simulink model "RHONN_EKF_FEEDBACK_FINAL_28_JULIO_2021"  (R2017b)
settings: Solver=ode1  StartTime=0.0  StopTime=60  FixedStep=0.001  RelTol=1e-3
model workspace (MATLAB code in the model file):
  | % ESTADOS INICIALES DE LOS ESTADOS X1, X2 Y X3
  | % Donde:
  | % x1 es representado con un vector de 3x1.
  | % x2 es representado con un vector de 2x1.
  | % x3 es representado con un vector de 2x1.
  | 
  | % Definir estados iniciales de las variables x11, x12 y x13 respectivamente.
  | init_x11 = 0;
  | init_x12 = 0;
  | init_x13 = 0;
  | % Estado inicial de x1
  | init_state_x1 = [init_x11; init_x12; init_x13];
  | 
  | % Definir estados iniciales de las variables x21 y x22 respectivamente.
  | init_x21 = 0.1;
  | init_x22 = 0.1;
  | % Estado inicial de x2
  | init_state_x2 = [init_x21; init_x22];
  | 
  | % Definir estados iniciales de las variables x31 y x32 respectivamente.
  | init_x31 = 0.1;
  | init_x32 = 0.1;
  | % Estado inicial de x3
  | init_state_x3 = [init_x31; init_x32];
  | 
  | % Definir el estado inicial de la ley de control U, representado por un vector de 2x1.
  | init_U1 = -1;
  | init_U2 = -1;
  | init_U = [init_U1; init_U2];
  | 
  | % INICIALIZACION DE VARIABLES >>>>>>>>>>>>>>>>>>>>>>>>>>>>>>>>
  | 
  |     %Constantes iniciales
  |     %La mitad del ancho del robot mobil.
  |     R = 0.75;
  |     %La distancia del centro de Pc del robot mobil a la mitad del punto medio
  |     %de P0 en medio de las ruedas izquierda y derecha.
  |     d = 0.3;
  |     %Radio de la rueda.
  |     r = 0.15;
  |     %Masa del cuerpo.
  |     mc = 30;
  |     %Masa de la rueda con motor.
  |     mw = 1;
  |     %Ic,Iw,Im son los momentos de inercia del cuerpo sobre el eje vertical a
  |     %traves de Pc.
  |     Ic = 15.625;
  |     Iw = 0.005;
  |     Im = 0.0025;
  |     %Resistencia.
  |     Ra = diag([2.5,2.5]);
  |     %Inductancia.
  |     La = diag([0.048,0.048]);
  |     %Coeficiente de fuera electromotriz trasero.
  |     KE = diag([0.02,0.02]);
  |     %Relacion de transmision.
  |     N = diag([62.55,62.55]);
  |     %Constante de torque del motor.
  |     KT = diag([0.2613,0.2613]);
  |     %d11, d12 son los coeficientes de amortiguamiento.
  |     d11 = 0.5;
  |     d12 = d11;
  |     %>>>>>>>>>>>>>>>>>>>>>>>>>>>>>>>>>>>>>>>>>>>>>>>>>>>>>>>><
  | 
  |     m = mc + (2 * mw);
  |     I = (mc * (d ^ 2)) + (2 * mw * (R^2)) + Ic + (2*Im);
  |     m11 = 0.25 * ( R ^ -2 ) * (r ^ 2) * ((m * (R ^ 2)) + I) + Iw;
  |     m12 = 0.25 * ( R ^ -2 ) * (r ^ 2) * ((m * (R ^ 2)) - I);
  |     M = [m11, m12; m12, m11];
  |     D = diag([d11, d12]);
  | 
  | 
  |  %VALORES HUERISTICOS SEGUN EL PAPER
  | %MODELO MATEMATICO
  | 
  | 
  | %Constantes iniciales
  | %La mitad del ancho del robot mobil.
  | R = 0.75;
  | %La distancia del centro de Pc del robot mobil a la mitad del punto medio
  | %de P0 en medio de las ruedas izquierda y derecha.
  | d = 0.3;
  | %Radio de la rueda.
  | r = 0.15;
  | %Masa del cuerpo.
  | mc = 30;
  | %Masa de la rueda con motor.
  | mw = 1;
  | %Ic,Iw,Im son los momentos de inercia del cuerpo sobre el eje vertical a
  | %traves de Pc.
  | Ic = 15.625;
  | Iw = 0.005;
  | Im = 0.0025;
  | %Resistencia.
  | Ra = diag([2.5,2.5]);
  | %Inductancia.
  | La = diag([0.048,0.048]);
  | %Coeficiente de fuera electromotriz trasero.
  | KE = diag([0.02,0.02]);
  | %Relacion de transmision.
  | N = diag([62.55,62.55]);
  | %Constante de torque del motor.
  | KT = diag([0.2613,0.2613]);
  | %d11, d12 son los coeficientes de amortiguamiento.
  | d11 = 0.5;
  | d12 = d11;
  | 
  | 
  | 
  | %NOTA : los valores cuya definicion se encuentre en minuscula
  | %se utiliza para generar de manera dinamica con programacion
  | %la variable final que se utiliza en el programa.
  | %De manera que si llegara a ser necesario solo se modificarian las variables iniciales
  | 
  | %VARIABLES INICIALES ========================================
  | 
  | p1 = 1 * (10^8);
  | p2 = 1 * (10^2);
  | p3 = 1 * (10^8);
  | p4 = 1 * (10^2);
  | p5 = 1 * (10^2);
  | p6 = 1 * (10^2);
  | p7 = 1 * (10^2);
  | 
  | r1 = 1 * (10^4);
  | r2 = 5 * (10^4);
  | r3 = 1 * (10^4);
  | r4 = 1 * (10^1);
  | r5 = 1 * (10^1);
  | r6 = 1 * (10^3);
  | r7 = 1 * (10^3);
  | 
  | q1 = 5 * (10^5);
  | q2 = 5 * (10^5);
  | q3 = 5 * (10^5);
  | q4 = 1 * (10^1);
  | q5 = 1 * (10^1);
  | q6 = 1 * (10^3);
  | q7 = 1 * (10^3);
  | 
  | G1 = 0.00001;
  | G2 = 0.00001;
  | 
  | %VALOREES INICIALES DE LOS PESOS USADOS EN EKF
  | 
  | %PESOS DE W1
  | W11 = 0.1;
  | W12 = 0.1;
  | %PESOS DE W2
  | W21 = 0.1;
  | W22 = 0.1;
  | %PESOS DE W3
  | W31 = 0.1;
  | W32 = 0.1;
  | %PESOS DE W4
  | W41 = 0.1;
  | W42 = 0.1;
  | W43 = 0.1;
  | W44 = 0.1;
  | %PESOS DE W5
  | W51 = 0.1;
  | W52 = 0.1;
  | W53 = 0.1;
  | W54 = 0.1;
  | %PESOS DE W6
  | W61 = 0.1;
  | W62 = 0.1;
  | W63 = 0.1;
  | W64 = 0.1;
  | %PESOS DE W7
  | W71 = 0.1;
  | W72 = 0.1;
  | W73 = 0.1;
  | W74 = 0.1;
  | 
  | %VALOR DE LAS SIGMOIDALES SUAVES
  | B = 2 * exp(-3);    %Este valor debe ser mayor a cero pero en base a mis observaciones menor a 1.
  | FO = 1;   %Este valor es obtenido de la tesis de la Dra Alma debe ser CERCANO y MENOR a 1, si este se vuelve 1 funcionara como FKE unicamente
  | 
  | 
  | %VARIABLES FINALES ========================================
  | 
  | %PARAMETROS DE ENTRENAMIENTO EKF PARA RHONN 1
  | W1 = [W11; W12]; %VALOR INICIAL de Vector de pesos para x1
  | P1 = diag([p1, p1]); %VALOR INICIAL de Matriz diagonal inicial de P1
  | R1 = r1; % Valor de R1
  | Q1 = diag([q1, q1]); % Valor de Q1
  | 
  | %PARAMETROS DE ENTRENAMIENTO EKF PARA RHONN 2
  | W2 = [W21; W22]; %VALOR INICIAL de Vector de pesos para x2
  | P2 = diag([p2, p2]); %VALOR INICIAL de Matriz diagonal inicial de P2
  | R2 = r2; % Valor de R2
  | Q2 = diag([q2, q2]); % Valor de Q2
  | 
  | %PARAMETROS DE ENTRENAMIENTO EKF PARA RHONN 3
  | W3 = [W31; W32]; %VALOR INICIAL de Vector de pesos para x3
  | P3 = diag([p3, p3]); %VALOR INICIAL de Matriz diagonal inicial de P3
  | R3 = r3; % Valor de R3
  | Q3 = diag([q3, q3]); % Valor de Q3
  | 
  | %PARAMETROS DE ENTRENAMIENTO EKF PARA RHONN 4
  | W4 = [W41; W42; W43; W44]; %VALOR INICIAL de Vector de pesos para x4
  | P4 = diag([p4, p4, p4, p4]); %VALOR INICIAL de Matriz diagonal inicial de P4
  | R4 = r4; % Valor de R4
  | Q4 = diag([q4, q4, q4, q4]); % Valor de Q4
  | 
  | %PARAMETROS DE ENTRENAMIENTO EKF PARA RHONN 5
  | W5 = [W51; W52; W53; W54]; %VALOR INICIAL de Vector de pesos para x5
  | P5 = diag([p5, p5, p5, p5]); %VALOR INICIAL de Matriz diagonal inicial de P5
  | R5 = r5; % Valor de R5
  | Q5 = diag([q5, q5, q5, q5]); % Valor de Q5
  | 
  | %PARAMETROS DE ENTRENAMIENTO EKF PARA RHONN 6
  | W6 = [W61; W62; W63; W64]; %VALOR INICIAL de Vector de pesos para x6
  | P6 = diag([p6, p6, p6, p6]); %VALOR INICIAL de Matriz diagonal inicial de P6
  | R6 = r6; % Valor de R6
  | Q6 = diag([q6, q6, q6, q6]); % Valor de Q6
  | 
  | %PARAMETROS DE ENTRENAMIENTO EKF PARA RHONN 7
  | W7 = [W71; W72; W73; W74]; %VALOR INICIAL de Vector de pesos para x7
  | P7 = diag([p7, p7, p7, p7]); %VALOR INICIAL de Matriz diagonal inicial de P7
  | R7 = r7; % Valor de R7
  | Q7 = diag([q7, q7, q7, q7]); % Valor de Q7
  | 
  | 
  | % PARAMETROS DEL CONTROL POR RETROALIMENTACION
  | % Donde K1 es representado con una matriz diagonal 3x3
  | % Donde K2 es representado con una matriz diagonal 2x2
  | % Donde K3 es representado con una matriz diagonal 2x2
  | 
  | % Ganancias individuales de la diagonal K1
  | k11 = 70;
  | k12 = k11;
  | k13 = k11;
  | 
  | % Ganancias individuales de la diagonal K2.
  | k21 = 50;
  | k22 = k21;
  | 
  | % Ganancias individuales de la diagonal K3.
  | k31 = 200;
  | k32 = k31;
  | 
  | % Matrices de gananciasK1, K2, K3.
  | K1 = diag([k11, k12, k13]);
  | K2 = diag([k21, k22]);
  | K3 = diag([k31, k32]);
libraries: simulink x5
(part 1 of 2)
settings Model: Creator=52324  LastModifiedBy=52324

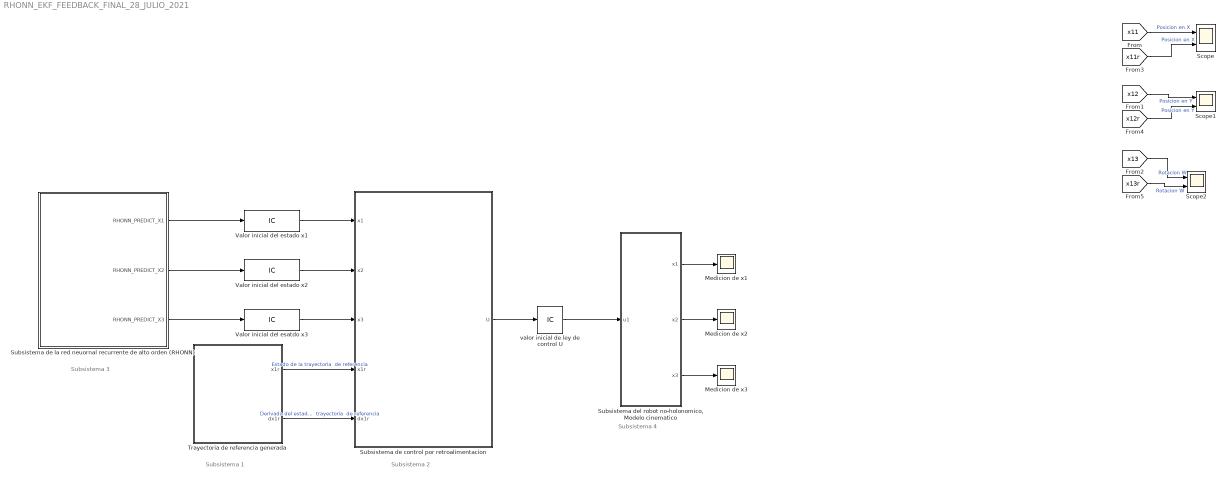
== system RHONN_EKF_FEEDBACK_FINAL_28_JULIO_2021 ==
  note: Subsistema 1
  note: Subsistema 2
  note: Subsistema 3
  note: Subsistema 4
  Medicion de x1 : Scope
  Medicion de x2 : Scope
  Medicion de x3 : Scope
  Scope : Scope  NumInputPorts=2
  Scope1 : Scope  NumInputPorts=2
  Scope2 : Scope  NumInputPorts=2
  Subsistema de control por retroalimentacion : Subsystem
  Subsistema de la red neuornal recurrente de alto orden (RHONN) : Subsystem
  "Subsistema del robot no-holonomico, Modelo cinematico" : Subsystem
  Trayectoria de referencia generada : Subsystem
  Valor inicial del esatdo x3 : InitialCondition  Value=init_state_x3
  Valor inicial del estado x1 : InitialCondition  Value=init_state_x1
  Valor inicial del estado x2 : InitialCondition  Value=init_state_x2
  valor inicial de ley de control U : InitialCondition  Value=init_U
  wires:
  [x11] -> Scope/1  "Posicion en X"
  [x11r] -> Scope/2  "Posicion en X"
  [x12] -> Scope1/1  "Posicion en Y"
  [x12r] -> Scope1/2  "Posicion en Y"
  [x13] -> Scope2/1  "Rotacion W"
  [x13r] -> Scope2/2  "Rotacion W"
  valor inicial de ley de control U/1 -> "Subsistema del robot no-holonomico, Modelo cinematico"/1(u1)
  "Subsistema del robot no-holonomico, Modelo cinematico"/1(x1) -> Medicion de x1/1
  Subsistema de la red neuornal recurrente de alto orden (RHONN)/1(RHONN_PREDICT_X1) -> Valor inicial del estado x1/1
  Subsistema de la red neuornal recurrente de alto orden (RHONN)/2(RHONN_PREDICT_X2) -> Valor inicial del estado x2/1
  Subsistema de la red neuornal recurrente de alto orden (RHONN)/3(RHONN_PREDICT_X3) -> Valor inicial del esatdo x3/1
  "Subsistema del robot no-holonomico, Modelo cinematico"/2(x2) -> Medicion de x2/1
  "Subsistema del robot no-holonomico, Modelo cinematico"/3(x3) -> Medicion de x3/1
  Subsistema de control por retroalimentacion/1(U) -> valor inicial de ley de control U/1
  Valor inicial del esatdo x3/1 -> Subsistema de control por retroalimentacion/3(x3)
  Valor inicial del estado x2/1 -> Subsistema de control por retroalimentacion/2(x2)
  Valor inicial del estado x1/1 -> Subsistema de control por retroalimentacion/1(x1)
  Trayectoria de referencia generada/1(x1r) -> Subsistema de control por retroalimentacion/4(x1r)  "Estado de la trayectoria  de referencia"
  Trayectoria de referencia generada/2(dx1r) -> Subsistema de control por retroalimentacion/5(dx1r)  "Derivada del estado de la  trayectoria  de referencia"

== system RHONN_EKF_FEEDBACK_FINAL_28_JULIO_2021/Subsistema de control por retroalimentacion ==
  note: Salida del subsistema
  x1 : Inport
  x2 : Inport  Port=2
  x3 : Inport  Port=3
  x1r : Inport  Port=4
  dx1r : Inport  Port=5
  Constant : Constant  Value=K1
  Constant1 : Constant  Value=K2
  Constant2 : Constant  Value=K3
  Derivative : Derivative
  MATLAB Function : MATLAB Function  TreatAsAtomicUnit=on
  Scope : Scope
  Scope2 : Scope
  Scope3 : Scope
  U : Outport
  wires:
  dx1r/1 -> MATLAB Function/4(dx1r)  "derivada del estado x1  de la trayectoria de referencia"
  x1r/1 -> MATLAB Function/2(x1r)  "estado x1  de la trayectoria de referencia"
  x1/1 -> MATLAB Function/1(x1)  "estado x1"
  x2/1 -> MATLAB Function/3(x2)  "estado x2"
  x3/1 -> MATLAB Function/7(x3)  "estado x3"
  MATLAB Function/4(U) -> U/1  "Ley de control U"
  [x13] -> Derivative/1, MATLAB Function/5(x13)
  Derivative/1 -> MATLAB Function/6(dx13)
  MATLAB Function/1(e1) -> Scope/1  "error 1"
  MATLAB Function/2(e2) -> Scope2/1  "error 2"
  MATLAB Function/3(e3) -> Scope3/1  "error 3"
  Constant/1 -> MATLAB Function/8(k1)  "Gnancia K1"
  Constant1/1 -> MATLAB Function/9(k2)  "Gnancia K2"
  Constant2/1 -> MATLAB Function/10(k3)  "Gnancia K3"

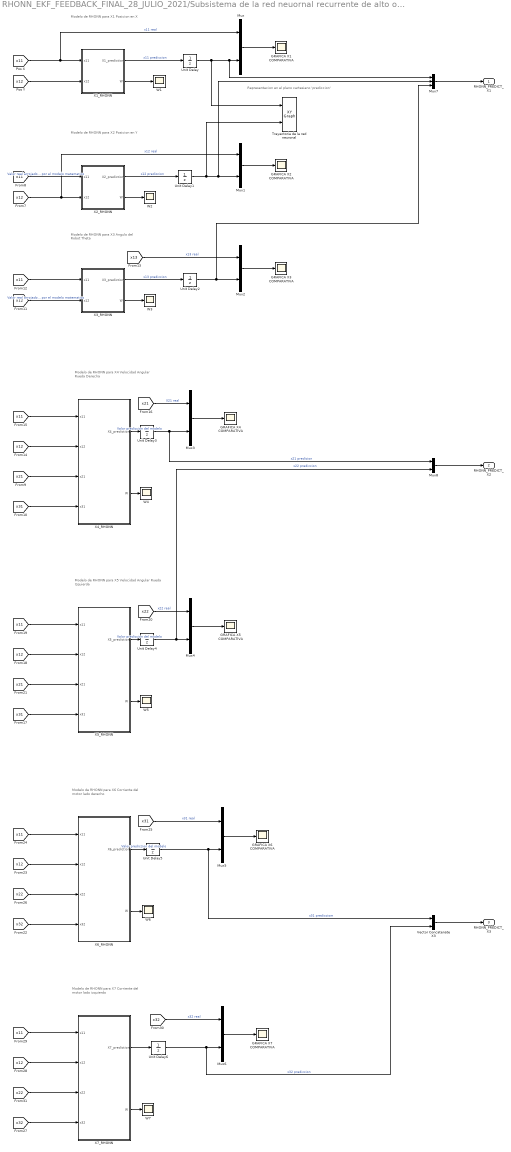
== system RHONN_EKF_FEEDBACK_FINAL_28_JULIO_2021/Subsistema de la red neuornal recurrente de alto orden (RHONN) ==
  note: Modelo de RHONN para X1
      | Posicion en X
  note: Modelo de RHONN para X5
      | Velocidad Angular Rueda Izquierda
  note: Modelo de RHONN para X2
      | Posicion en Y
  note: Modelo de RHONN para X3
      | Angulo del Robot Theta
  note: Modelo de RHONN para X4
      | Velocidad Angular Rueda Derecha
  note: Representacion en el plano cartesiano 'prediccion'
  note: Modelo de RHONN para X6
      | Corriente del motor lado derecho
  note: Modelo de RHONN para X7
      | Corriente del motor lado izquierdo
  GRAFICA X1 COMPARATIVA : Scope
  GRAFICA X2 COMPARATIVA : Scope
  GRAFICA X3 COMPARATIVA : Scope
  GRAFICA X4 COMPARATIVA : Scope
  GRAFICA X5 COMPARATIVA : Scope
  GRAFICA X6 COMPARATIVA : Scope
  GRAFICA X7 COMPARATIVA : Scope
  Mux{,1..6,8} (8 alike) : Mux  Inputs=2
  Mux7 : Mux  Inputs=3
  Trayectoria de la red neuronal : simulink/Sinks/XY Graph  xmin=-2.5  xmax=2.5  ymin=-2.5  ymax=2.5  st=-1
  Unit Delay : UnitDelay  InitialCondition=init_x11  SampleTime=-1
  Unit Delay1 : UnitDelay  InitialCondition=init_x12  SampleTime=-1
  Unit Delay2 : UnitDelay  InitialCondition=init_x13  SampleTime=-1
  Unit Delay3 : UnitDelay  InitialCondition=init_x21  SampleTime=-1
  Unit Delay4 : UnitDelay  InitialCondition=init_x22  SampleTime=-1
  Unit Delay5 : UnitDelay  InitialCondition=init_x31  SampleTime=-1
  Unit Delay6 : UnitDelay  InitialCondition=init_x32  SampleTime=-1
  Vector Concatenate X3 : Concatenate
  W{1..7} (7 alike) : Scope
  X1_RHONN : Subsystem
  X2_RHONN : Subsystem
  X3_RHONN : Subsystem
  X4_RHONN : Subsystem
  X5_RHONN : Subsystem
  X6_RHONN : Subsystem
  X7_RHONN : Subsystem
  RHONN_PREDICT_X1 : Outport
  RHONN_PREDICT_X2 : Outport  Port=2
  RHONN_PREDICT_X3 : Outport  Port=3
  wires:
  X6_RHONN/1(X6_prediction) -> Unit Delay5/1  "Valor prediccion del modelo"
  [x12] -> X5_RHONN/2(x12)
  X2_RHONN/1(X2_prediction) -> Unit Delay1/1  "x12 prediccion"
  [x12] -> X7_RHONN/2(x12)
  X1_RHONN/2(W) -> W1/1
  [x12] -> Mux1/1, X2_RHONN/2(x12)  "x12 real"
  X5_RHONN/2(W) -> W5/1
  Mux4/1 -> GRAFICA X5 COMPARATIVA/1
  X6_RHONN/2(W) -> W6/1
  [x11] -> X6_RHONN/1(x11)
  [x31] -> Mux5/1  "x31 real"
  [x22] -> X7_RHONN/3(x22)
  [x11] -> X2_RHONN/1(x11)  "Valor real arrojado por el modelo matematico"
  X4_RHONN/2(W) -> W4/1
  [x11] -> X7_RHONN/1(x11)
  X7_RHONN/1(X7_prediction) -> Unit Delay6/1
  X3_RHONN/2(W) -> W3/1
  Mux3/1 -> GRAFICA X4 COMPARATIVA/1
  Mux6/1 -> GRAFICA X7 COMPARATIVA/1
  [x13] -> Mux2/1  "x13 real"
  [x11] -> X5_RHONN/1(x11)
  X5_RHONN/1(X5_prediction) -> Unit Delay4/1  "Valor prediccion del modelo"
  [x21] -> Mux3/1  "X21 real"
  Mux2/1 -> GRAFICA X3 COMPARATIVA/1
  [x32] -> X7_RHONN/4(x32)
  [x22] -> Mux4/1  "x22 real"
  Mux/1 -> GRAFICA X1 COMPARATIVA/1
  [x21] -> X5_RHONN/3(x21)
  [x11] -> X4_RHONN/1(x11)
  X4_RHONN/1(X4_prediction) -> Unit Delay3/1  "Valor prediccion del modelo"
  Mux5/1 -> GRAFICA X6 COMPARATIVA/1
  [x21] -> X4_RHONN/3(x21)
  X2_RHONN/2(W) -> W2/1
  X7_RHONN/2(W) -> W7/1
  [x12] -> X6_RHONN/2(x12)
  Mux1/1 -> GRAFICA X2 COMPARATIVA/1
  [x31] -> X5_RHONN/4(x31)
  [x22] -> X6_RHONN/3(x22)
  [x11] -> Mux/1, X1_RHONN/1(x11)  "x11 real"
  [x12] -> X4_RHONN/2(x12)
  X1_RHONN/1(X1_prediction) -> Unit Delay/1  "x11 prediccion"
  [x32] -> Mux6/1  "x32 real"
  [x31] -> X4_RHONN/4(x31)
  [x12] -> X3_RHONN/2(x12)  "Valor real arrojado por el modelo matematico"
  X3_RHONN/1(X3_prediction) -> Unit Delay2/1  "x13 prediccion"
  [x32] -> X6_RHONN/4(x32)
  Mux7/1 -> RHONN_PREDICT_X1/1
  Mux8/1 -> RHONN_PREDICT_X2/1
  Vector Concatenate X3/1 -> RHONN_PREDICT_X3/1
  [x12] -> X1_RHONN/2(x12)
  [x11] -> X3_RHONN/1(x11)
  Unit Delay/1 -> Trayectoria de la red neuronal/1, Mux7/1, Mux/2
  Unit Delay1/1 -> Trayectoria de la red neuronal/2, Mux7/2, Mux1/2
  Unit Delay2/1 -> Mux7/3, Mux2/2
  Unit Delay3/1 -> Mux8/1, Mux3/2  "x21 predicion"
  Unit Delay4/1 -> Mux8/2, Mux4/2  "x22 prediccion"
  Unit Delay5/1 -> Vector Concatenate X3/1, Mux5/2  "x31 predicciom"
  Unit Delay6/1 -> Vector Concatenate X3/2, Mux6/2  "x32 prediccion"

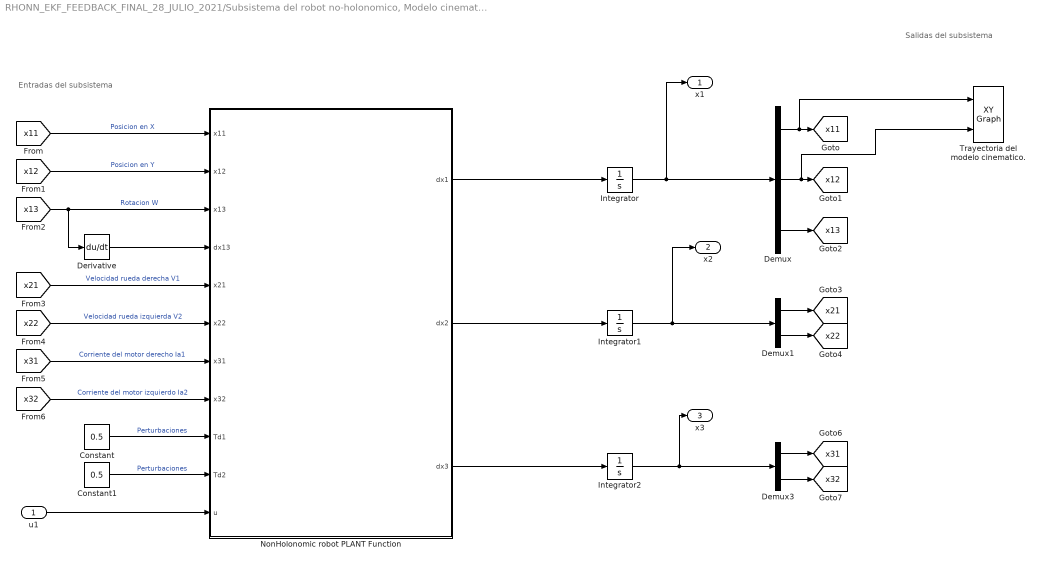
== system RHONN_EKF_FEEDBACK_FINAL_28_JULIO_2021/Subsistema del robot no-holonomico, Modelo cinematico ==
  note: Salidas del subsistema
  note: Entradas del subsistema
  u1 : Inport
  Constant : Constant  Value=0.5
  Constant1 : Constant  Value=0.5
  Demux : Demux  Outputs=3
  Demux1 : Demux  Outputs=2
  Demux3 : Demux  Outputs=2
  Derivative : Derivative
  Integrator : Integrator  InitialCondition=[0.1;0.1;0.1]
  Integrator1 : Integrator  InitialCondition=[0.1;0.1]
  Integrator2 : Integrator  InitialCondition=[0.1;0.1]
  NonHolonomic robot PLANT Function : MATLAB Function  TreatAsAtomicUnit=on
  Trayectoria del modelo cinematico. : simulink/Sinks/XY Graph  xmin=-2.5  xmax=2.5  ymin=-2.5  ymax=2.5  st=-1
  x1 : Outport
  x2 : Outport  Port=2
  x3 : Outport  Port=3
  tag scope: x11=global, x12=global, x13=global, x21=global, x22=global, x31=global, x32=global
  wires:
  [x31] -> NonHolonomic robot PLANT Function/7(x31)  "Corriente del motor derecho Ia1"
  NonHolonomic robot PLANT Function/2(dx2) -> Integrator1/1
  [x21] -> NonHolonomic robot PLANT Function/5(x21)  "Velocidad rueda derecha V1"
  Integrator1/1 -> x2/1, Demux1/1
  Constant1/1 -> NonHolonomic robot PLANT Function/10(Td2)  "Perturbaciones"
  [x12] -> NonHolonomic robot PLANT Function/2(x12)  "Posicion en Y"
  Derivative/1 -> NonHolonomic robot PLANT Function/4(dx13)
  Demux1/2 -> [x22]
  [x22] -> NonHolonomic robot PLANT Function/6(x22)  "Velocidad rueda izquierda V2"
  Demux3/1 -> [x31]
  Demux/3 -> [x13]
  [x11] -> NonHolonomic robot PLANT Function/1(x11)  "Posicion en X"
  Constant/1 -> NonHolonomic robot PLANT Function/9(Td1)  "Perturbaciones"
  [x32] -> NonHolonomic robot PLANT Function/8(x32)  "Corriente del motor izquierdo Ia2"
  Demux/1 -> Trayectoria del modelo cinematico./1, [x11]
  Demux1/1 -> [x21]
  Demux3/2 -> [x32]
  Integrator2/1 -> x3/1, Demux3/1
  Demux/2 -> Trayectoria del modelo cinematico./2, [x12]
  [x13] -> NonHolonomic robot PLANT Function/3(x13), Derivative/1  "Rotacion W"
  NonHolonomic robot PLANT Function/3(dx3) -> Integrator2/1
  NonHolonomic robot PLANT Function/1(dx1) -> Integrator/1
  u1/1 -> NonHolonomic robot PLANT Function/11(u)
  Integrator/1 -> x1/1, Demux/1

== system RHONN_EKF_FEEDBACK_FINAL_28_JULIO_2021/Trayectoria de referencia generada ==
  note: Salidas del subsistema
  note: Entrada del subsistema
  Constant : Constant
  Constant1 : Constant
  Demux : Demux  Outputs=3
  Demux1 : Demux  Outputs=3
  Derivative : Derivative
  Integrator3 : Integrator  InitialCondition=[0.1;0.1;0.1]
  Reference robot function : MATLAB Function  TreatAsAtomicUnit=on
  Trayectoria de referencia : simulink/Sinks/XY Graph  xmin=-2.5  xmax=2.5  ymin=-2.5  ymax=2.5  st=-1
  angulo de referencia : Scope
  x1r : Outport
  dx1r : Outport  Port=2
  tag scope: x11r=global, x12r=global, x13r=global
  wires:
  Demux/2 -> Trayectoria de referencia/2
  Reference robot function/1(dx1r) -> Integrator3/1
  Integrator3/1 -> Demux1/1, x1r/1, Derivative/1, Demux/1
  Demux/1 -> Trayectoria de referencia/1
  Constant/1 -> Reference robot function/1(Vr)
  Constant1/1 -> Reference robot function/2(Wr)
  Demux1/2 -> [x12r]
  Demux1/1 -> [x11r]
  Demux1/3 -> [x13r]
  [x13r] -> Reference robot function/3(Or)
  Demux/3 -> angulo de referencia/1
  Derivative/1 -> dx1r/1

== system RHONN_EKF_FEEDBACK_FINAL_28_JULIO_2021/Subsistema de la red neuornal recurrente de alto orden (RHONN)/X1_RHONN ==
  note: Filtro extendido de kalman (EKF)
  note: Funcion RHONN
      |
      | X(k+1) = w11 * S(x11) + w12 * S(x12)
  x11 : Inport
  x12 : Inport  Port=2
  Generador de matriz H : MATLAB Function  TreatAsAtomicUnit=on
  Sigmoidal suave1 : Subsystem
  Sigmoidal suave3 : Subsystem
  X1_EKF : Subsystem
  X1_RHONN : MATLAB Function  TreatAsAtomicUnit=on
  X1_prediction : Outport
  W : Outport  Port=2
  wires:
  X1_RHONN/1(pred) -> X1_EKF/2(prediccion), X1_prediction/1  "Valor predicho por la red neuronal"
  Sigmoidal suave3/1(salida) -> Generador de matriz H/2(Sx12), X1_RHONN/3(Sx12)  "S(x12)"
  x12/1 -> Sigmoidal suave3/1(c)
  x11/1 -> X1_EKF/1(medicion), Sigmoidal suave1/1(c)
  Sigmoidal suave1/1(salida) -> Generador de matriz H/1(Sx11), X1_RHONN/2(Sx11)  "S(x11)"
  Generador de matriz H/1(H) -> X1_EKF/3(H)  "Valor de matriz H"
  X1_EKF/1(W) -> W/1, X1_RHONN/1(W)  "Valor actualizado de los pesos"

== system RHONN_EKF_FEEDBACK_FINAL_28_JULIO_2021/Subsistema de la red neuornal recurrente de alto orden (RHONN)/X2_RHONN ==
  note: Filtro extendido de kalman (EKF)
  note: Funcion RHONN
      |
      | X2(k+1) = w21 * S(x11) + w22 * S(x12)
  x11 : Inport
  x12 : Inport  Port=2
  Generador de matriz H : MATLAB Function  TreatAsAtomicUnit=on
  Sigmoidal suave1 : Subsystem
  Sigmoidal suave3 : Subsystem
  X2_EKF : Subsystem
  X2_RHONN_function : MATLAB Function  TreatAsAtomicUnit=on
  X2_prediction : Outport
  W : Outport  Port=2
  wires:
  X2_RHONN_function/1(pred) -> X2_EKF/2(prediccion), X2_prediction/1  "Valor predicho por la red neuronal"
  Sigmoidal suave3/1(salida) -> Generador de matriz H/2(Sx12), X2_RHONN_function/3(Sx12)  "S(x12)"
  x12/1 -> X2_EKF/1(medicion), Sigmoidal suave3/1(c)
  x11/1 -> Sigmoidal suave1/1(c)
  Sigmoidal suave1/1(salida) -> Generador de matriz H/1(Sx11), X2_RHONN_function/2(Sx11)  "S(x11)"
  Generador de matriz H/1(H) -> X2_EKF/3(H)  "Valor de matriz H"
  X2_EKF/1(W) -> X2_RHONN_function/1(W), W/1  "Valor actualizado de los pesos"

== system RHONN_EKF_FEEDBACK_FINAL_28_JULIO_2021/Subsistema de la red neuornal recurrente de alto orden (RHONN)/X3_RHONN ==
  note: Para este caso el error debe ser basado a la medicion del angulo del robot (x13)
  note: Filtro extendido de kalman (EKF)
  note: Funcion RHONN
      |
      | X3(k+1) = w31 * S(x11) + w32 * S(x12)
  x11 : Inport
  x12 : Inport  Port=2
  Generador de matriz H : MATLAB Function  TreatAsAtomicUnit=on
  Sigmoidal suave1 : Subsystem
  Sigmoidal suave3 : Subsystem
  X3_EKF : Subsystem
  X3_RHONN_function : MATLAB Function  TreatAsAtomicUnit=on
  X3_prediction : Outport
  W : Outport  Port=2
  wires:
  X3_RHONN_function/1(pred) -> X3_EKF/2(prediccion), X3_prediction/1  "Valor predicho por la red neuronal"
  Sigmoidal suave3/1(salida) -> Generador de matriz H/2(Sx12), X3_RHONN_function/3(Sx12)  "S(x12)"
  x12/1 -> Sigmoidal suave3/1(c)
  x11/1 -> Sigmoidal suave1/1(c)
  Sigmoidal suave1/1(salida) -> Generador de matriz H/1(Sx11), X3_RHONN_function/2(Sx11)  "S(x11)"
  Generador de matriz H/1(H) -> X3_EKF/3(H)  "Valor de matriz H"
  X3_EKF/1(W) -> W/1, X3_RHONN_function/1(W)  "Valor actualizado de los pesos"
  [x13] -> X3_EKF/1(medicion)  "Angulo del robot medido"

== system RHONN_EKF_FEEDBACK_FINAL_28_JULIO_2021/Subsistema de la red neuornal recurrente de alto orden (RHONN)/X4_RHONN ==
  note: Para este caso el error debe ser basado a la medicion de la velocidad angular de la rueda derecha (x21)
  note: Filtro extendido de kalman (EKF)
  note: Funcion RHONN
      |
      | X4(k+1) = w41 * S(x11) + w42 * S(x12) + w43*S(x21) + w44*S(x31)
  x11 : Inport
  x12 : Inport  Port=2
  x21 : Inport  Port=3
  x31 : Inport  Port=4
  Generador de matriz H : MATLAB Function  TreatAsAtomicUnit=on
  Sigmoidal suave1 : Subsystem
  Sigmoidal suave2 : Subsystem
  Sigmoidal suave3 : Subsystem
  Sigmoidal suave4 : Subsystem
  X4_EKF : Subsystem
  X4_RHONN_function : MATLAB Function  TreatAsAtomicUnit=on
  X4_prediction : Outport
  W : Outport  Port=2
  wires:
  X4_RHONN_function/1(pred) -> X4_EKF/2(prediccion), X4_prediction/1  "Valor predicho por la red neuronal"
  Sigmoidal suave3/1(salida) -> Generador de matriz H/2(Sx12), X4_RHONN_function/3(Sx12)  "S(x12)"
  x12/1 -> Sigmoidal suave3/1(c)
  x11/1 -> Sigmoidal suave1/1(c)
  Sigmoidal suave1/1(salida) -> Generador de matriz H/1(Sx11), X4_RHONN_function/2(Sx11)  "S(x11)"
  Generador de matriz H/1(H) -> X4_EKF/3(H)  "Valor de matriz H"
  X4_EKF/1(W) -> X4_RHONN_function/1(W), W/1  "Valor actualizado de los pesos"
  [x21] -> X4_EKF/1(medicion)  "Angulo del robot medido"
  x21/1 -> Sigmoidal suave2/1(c)
  x31/1 -> Sigmoidal suave4/1(c)
  Sigmoidal suave2/1(salida) -> Generador de matriz H/3(Sx21), X4_RHONN_function/4(Sx21)  "S(x21)"
  Sigmoidal suave4/1(salida) -> Generador de matriz H/4(Sx31), X4_RHONN_function/5(Sx31)  "S(x31)"

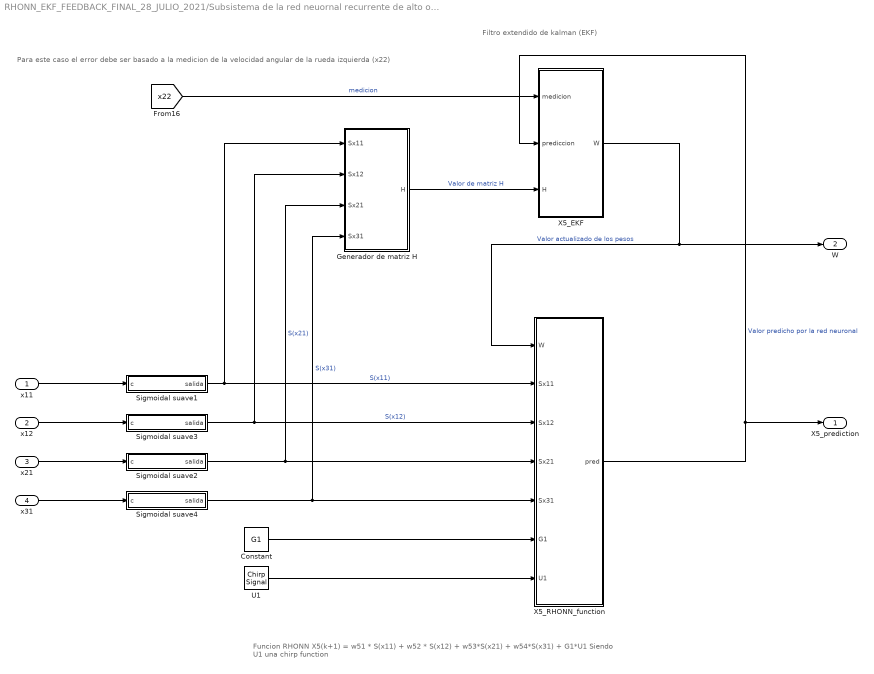
== system RHONN_EKF_FEEDBACK_FINAL_28_JULIO_2021/Subsistema de la red neuornal recurrente de alto orden (RHONN)/X5_RHONN ==
  note: Para este caso el error debe ser basado a la medicion de la velocidad angular de la rueda izquierda (x22)
  note: Filtro extendido de kalman (EKF)
  note: Funcion RHONN
      |
      | X5(k+1) = w51 * S(x11) + w52 * S(x12) + w53*S(x21) + w54*S(x31) + G1*U1
      |
      | Siendo U1 una chirp function
  x11 : Inport
  x12 : Inport  Port=2
  x21 : Inport  Port=3
  x31 : Inport  Port=4
  Constant : Constant  Value=G1
  Generador de matriz H : MATLAB Function  TreatAsAtomicUnit=on
  Sigmoidal suave1 : Subsystem
  Sigmoidal suave2 : Subsystem
  Sigmoidal suave3 : Subsystem
  Sigmoidal suave4 : Subsystem
  U1 : simulink/Sources/Chirp Signal  f1=0.1  T=100  f2=1
  X5_EKF : Subsystem
  X5_RHONN_function : MATLAB Function  TreatAsAtomicUnit=on
  X5_prediction : Outport
  W : Outport  Port=2
  wires:
  X5_RHONN_function/1(pred) -> X5_EKF/2(prediccion), X5_prediction/1  "Valor predicho por la red neuronal"
  Sigmoidal suave3/1(salida) -> Generador de matriz H/2(Sx12), X5_RHONN_function/3(Sx12)  "S(x12)"
  x12/1 -> Sigmoidal suave3/1(c)
  x11/1 -> Sigmoidal suave1/1(c)
  Sigmoidal suave1/1(salida) -> Generador de matriz H/1(Sx11), X5_RHONN_function/2(Sx11)  "S(x11)"
  Generador de matriz H/1(H) -> X5_EKF/3(H)  "Valor de matriz H"
  X5_EKF/1(W) -> W/1, X5_RHONN_function/1(W)  "Valor actualizado de los pesos"
  [x22] -> X5_EKF/1(medicion)  "medicion"
  x21/1 -> Sigmoidal suave2/1(c)
  x31/1 -> Sigmoidal suave4/1(c)
  Sigmoidal suave2/1(salida) -> Generador de matriz H/3(Sx21), X5_RHONN_function/4(Sx21)  "S(x21)"
  Sigmoidal suave4/1(salida) -> Generador de matriz H/4(Sx31), X5_RHONN_function/5(Sx31)  "S(x31)"
  Constant/1 -> X5_RHONN_function/6(G1)
  U1/1 -> X5_RHONN_function/7(U1)

== system RHONN_EKF_FEEDBACK_FINAL_28_JULIO_2021/Subsistema de la red neuornal recurrente de alto orden (RHONN)/X6_RHONN ==
  note: Para este caso el error debe ser basado a la medicion de la corriente de la rueda derecha (x31)
  note: Filtro extendido de kalman (EKF)
  note: Funcion RHONN
      |
      | X6(k+1) = w61 * S(x11) + w62 * S(x12) + w63*S(x22) + w64*S(x32)
  x11 : Inport
  x12 : Inport  Port=2
  x22 : Inport  Port=3
  x32 : Inport  Port=4
  Generador de matriz H : MATLAB Function  TreatAsAtomicUnit=on
  Sigmoidal suave1 : Subsystem
  Sigmoidal suave2 : Subsystem
  Sigmoidal suave3 : Subsystem
  Sigmoidal suave4 : Subsystem
  X6_EKF : Subsystem
  X6_RHONN_function : MATLAB Function  TreatAsAtomicUnit=on
  X6_prediction : Outport
  W : Outport  Port=2
  wires:
  X6_RHONN_function/1(pred) -> X6_EKF/2(prediccion), X6_prediction/1  "Valor predicho por la red neuronal"
  Sigmoidal suave3/1(salida) -> Generador de matriz H/2(Sx12), X6_RHONN_function/3(Sx12)  "S(x12)"
  x12/1 -> Sigmoidal suave3/1(c)
  x11/1 -> Sigmoidal suave1/1(c)
  Sigmoidal suave1/1(salida) -> Generador de matriz H/1(Sx11), X6_RHONN_function/2(Sx11)  "S(x11)"
  Generador de matriz H/1(H) -> X6_EKF/3(H)  "Valor de matriz H"
  X6_EKF/1(W) -> W/1, X6_RHONN_function/1(W)  "Valor actualizado de los pesos"
  [x31] -> X6_EKF/1(medicion)  "medicion"
  x22/1 -> Sigmoidal suave2/1(c)
  x32/1 -> Sigmoidal suave4/1(c)
  Sigmoidal suave2/1(salida) -> Generador de matriz H/3(Sx22), X6_RHONN_function/4(Sx22)  "S(x22)"
  Sigmoidal suave4/1(salida) -> Generador de matriz H/4(Sx32), X6_RHONN_function/5(Sx32)  "S(x32)"

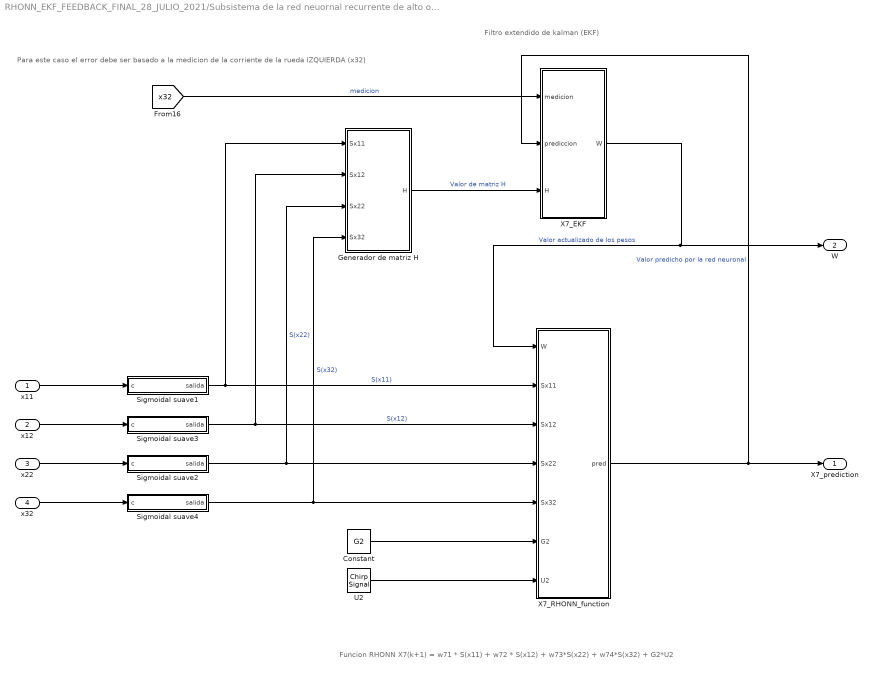
== system RHONN_EKF_FEEDBACK_FINAL_28_JULIO_2021/Subsistema de la red neuornal recurrente de alto orden (RHONN)/X7_RHONN ==
  note: Para este caso el error debe ser basado a la medicion de la corriente de la rueda IZQUIERDA (x32)
  note: Filtro extendido de kalman (EKF)
  note: Funcion RHONN
      |
      | X7(k+1) = w71 * S(x11) + w72 * S(x12) + w73*S(x22) + w74*S(x32) + G2*U2
  x11 : Inport
  x12 : Inport  Port=2
  x22 : Inport  Port=3
  x32 : Inport  Port=4
  Constant : Constant  Value=G2
  Generador de matriz H : MATLAB Function  TreatAsAtomicUnit=on
  Sigmoidal suave1 : Subsystem
  Sigmoidal suave2 : Subsystem
  Sigmoidal suave3 : Subsystem
  Sigmoidal suave4 : Subsystem
  U2 : simulink/Sources/Chirp Signal  f1=0.1  T=100  f2=1
  X7_EKF : Subsystem
  X7_RHONN_function : MATLAB Function  TreatAsAtomicUnit=on
  X7_prediction : Outport
  W : Outport  Port=2
  wires:
  X7_RHONN_function/1(pred) -> X7_EKF/2(prediccion), X7_prediction/1  "Valor predicho por la red neuronal"
  Sigmoidal suave3/1(salida) -> Generador de matriz H/2(Sx12), X7_RHONN_function/3(Sx12)  "S(x12)"
  x12/1 -> Sigmoidal suave3/1(c)
  x11/1 -> Sigmoidal suave1/1(c)
  Sigmoidal suave1/1(salida) -> Generador de matriz H/1(Sx11), X7_RHONN_function/2(Sx11)  "S(x11)"
  Generador de matriz H/1(H) -> X7_EKF/3(H)  "Valor de matriz H"
  X7_EKF/1(W) -> W/1, X7_RHONN_function/1(W)  "Valor actualizado de los pesos"
  [x32] -> X7_EKF/1(medicion)  "medicion"
  x22/1 -> Sigmoidal suave2/1(c)
  x32/1 -> Sigmoidal suave4/1(c)
  Sigmoidal suave2/1(salida) -> Generador de matriz H/3(Sx22), X7_RHONN_function/4(Sx22)  "S(x22)"
  Sigmoidal suave4/1(salida) -> Generador de matriz H/4(Sx32), X7_RHONN_function/5(Sx32)  "S(x32)"
  Constant/1 -> X7_RHONN_function/6(G2)
  U2/1 -> X7_RHONN_function/7(U2)

== system RHONN_EKF_FEEDBACK_FINAL_28_JULIO_2021/Subsistema de la red neuornal recurrente de alto orden (RHONN)/X1_RHONN/Sigmoidal suave1 ==
  note: Funcion sigmoidal suave S(*)
  note: Dada la ecuacion (5) del paper:
      | B > 0
      |
      | Y observado en la tesis de la Dra Alma
      | B = 2e^-3
  c : Inport
  Constante de sigmoidal suave : Constant  Value=B
  Sigmoidal suave : MATLAB Function  TreatAsAtomicUnit=on
  salida : Outport
  wires:
  Sigmoidal suave/1(sig) -> salida/1  "Señal transformada S(*)"
  c/1 -> Sigmoidal suave/2(c)  "Señal a transformar"
  Constante de sigmoidal suave/1 -> Sigmoidal suave/1(B)

== system RHONN_EKF_FEEDBACK_FINAL_28_JULIO_2021/Subsistema de la red neuornal recurrente de alto orden (RHONN)/X1_RHONN/Sigmoidal suave3 ==
  note: Funcion sigmoidal suave S(*)
  note: Dada la ecuacion (5) del paper:
      | B > 0
      |
      | Y observado en la tesis de la Dra Alma
      | B = 2e^-3
  c : Inport
  Constante de sigmoidal suave : Constant  Value=B
  Sigmoidal suave : MATLAB Function  TreatAsAtomicUnit=on
  salida : Outport
  wires:
  Sigmoidal suave/1(sig) -> salida/1  "Señal transformada S(*)"
  c/1 -> Sigmoidal suave/2(c)  "Señal a transformar"
  Constante de sigmoidal suave/1 -> Sigmoidal suave/1(B)

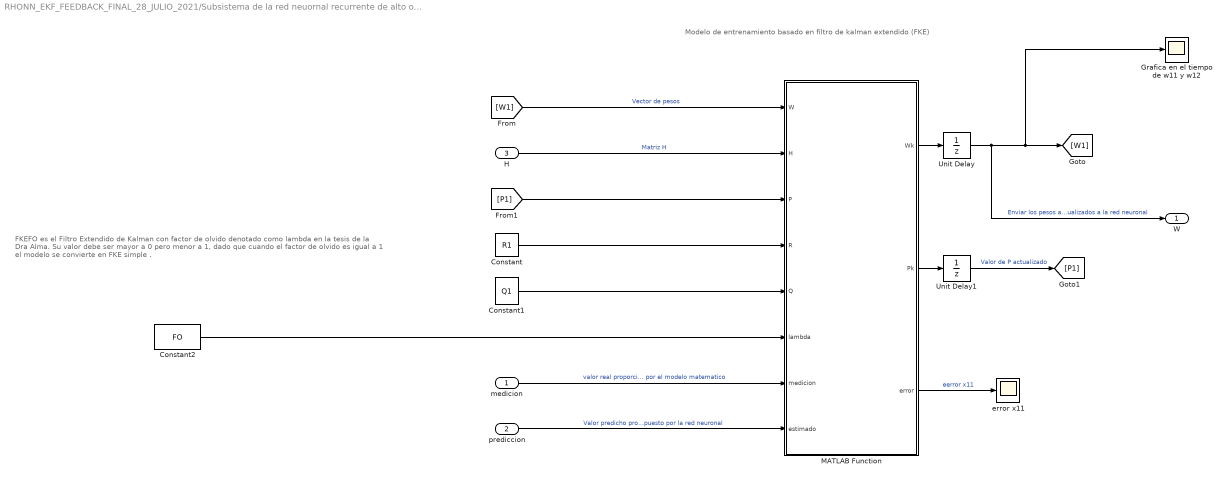
== system RHONN_EKF_FEEDBACK_FINAL_28_JULIO_2021/Subsistema de la red neuornal recurrente de alto orden (RHONN)/X1_RHONN/X1_EKF ==
  note: FKEFO es el Filtro Extendido de Kalman con factor de olvido
      |
      | denotado como lambda en la tesis de la Dra Alma.
      | Su valor debe ser mayor a 0 pero menor a 1, dado que cuando
      | el factor de olvido es igual a 1 el modelo se convierte en FKE simple .
  note: Modelo de entrenamiento basado en filtro de kalman extendido (FKE)
  medicion : Inport
  prediccion : Inport  Port=2
  H : Inport  Port=3
  Constant : Constant  Value=R1
  Constant1 : Constant  Value=Q1
  Constant2 : Constant  Value=FO
  Grafica en el tiempo de w11 y w12 : Scope
  MATLAB Function : MATLAB Function  TreatAsAtomicUnit=on
  Unit Delay : UnitDelay  InitialCondition=W1  SampleTime=-1
  Unit Delay1 : UnitDelay  InitialCondition=P1  SampleTime=-1
  error x11 : Scope
  W : Outport
  wires:
  prediccion/1 -> MATLAB Function/8(estimado)  "Valor predicho propuesto por la red neuronal"
  medicion/1 -> MATLAB Function/7(medicion)  "valor real proporcionado por el modelo matematico"
  MATLAB Function/1(Wk) -> Unit Delay/1
  [W1] -> MATLAB Function/1(W)  "Vector de pesos"
  MATLAB Function/2(Pk) -> Unit Delay1/1
  [P1] -> MATLAB Function/3(P)
  Constant/1 -> MATLAB Function/4(R)
  Constant1/1 -> MATLAB Function/5(Q)
  H/1 -> MATLAB Function/2(H)  "Matriz H"
  Unit Delay1/1 -> [P1]  "Valor de P actualizado"
  Unit Delay/1 -> Grafica en el tiempo de w11 y w12/1, [W1], W/1  "Enviar los pesos actualizados a la red neuronal"
  Constant2/1 -> MATLAB Function/6(lambda)
  MATLAB Function/3(error) -> error x11/1  "eerror x11"

== system RHONN_EKF_FEEDBACK_FINAL_28_JULIO_2021/Subsistema de la red neuornal recurrente de alto orden (RHONN)/X2_RHONN/Sigmoidal suave1 ==
  note: Funcion sigmoidal suave S(*)
  note: Dada la ecuacion (5) del paper:
      | B > 0
      |
      | Y observado en la tesis de la Dra Alma
      | B = 2e^-3
  c : Inport
  Constante de sigmoidal suave : Constant  Value=B
  Sigmoidal suave : MATLAB Function  TreatAsAtomicUnit=on
  salida : Outport
  wires:
  Sigmoidal suave/1(sig) -> salida/1  "Señal transformada S(*)"
  c/1 -> Sigmoidal suave/2(c)  "Señal a transformar"
  Constante de sigmoidal suave/1 -> Sigmoidal suave/1(B)

== system RHONN_EKF_FEEDBACK_FINAL_28_JULIO_2021/Subsistema de la red neuornal recurrente de alto orden (RHONN)/X2_RHONN/Sigmoidal suave3 ==
  note: Funcion sigmoidal suave S(*)
  note: Dada la ecuacion (5) del paper:
      | B > 0
      |
      | Y observado en la tesis de la Dra Alma
      | B = 2e^-3
  c : Inport
  Constante de sigmoidal suave : Constant  Value=B
  Sigmoidal suave : MATLAB Function  TreatAsAtomicUnit=on
  salida : Outport
  wires:
  Sigmoidal suave/1(sig) -> salida/1  "Señal transformada S(*)"
  c/1 -> Sigmoidal suave/2(c)  "Señal a transformar"
  Constante de sigmoidal suave/1 -> Sigmoidal suave/1(B)

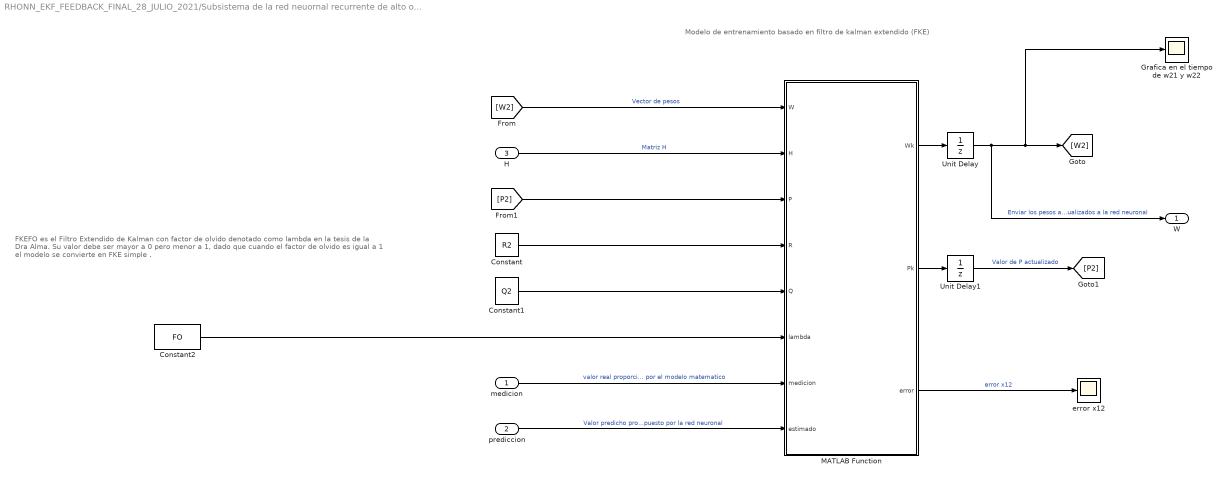
== system RHONN_EKF_FEEDBACK_FINAL_28_JULIO_2021/Subsistema de la red neuornal recurrente de alto orden (RHONN)/X2_RHONN/X2_EKF ==
  note: FKEFO es el Filtro Extendido de Kalman con factor de olvido
      |
      | denotado como lambda en la tesis de la Dra Alma.
      | Su valor debe ser mayor a 0 pero menor a 1, dado que cuando
      | el factor de olvido es igual a 1 el modelo se convierte en FKE simple .
  note: Modelo de entrenamiento basado en filtro de kalman extendido (FKE)
  medicion : Inport
  prediccion : Inport  Port=2
  H : Inport  Port=3
  Constant : Constant  Value=R2
  Constant1 : Constant  Value=Q2
  Constant2 : Constant  Value=FO
  Grafica en el tiempo de w21 y w22 : Scope
  MATLAB Function : MATLAB Function  TreatAsAtomicUnit=on
  Unit Delay : UnitDelay  InitialCondition=W2  SampleTime=-1
  Unit Delay1 : UnitDelay  InitialCondition=P2  SampleTime=-1
  error x12 : Scope
  W : Outport
  wires:
  prediccion/1 -> MATLAB Function/8(estimado)  "Valor predicho propuesto por la red neuronal"
  medicion/1 -> MATLAB Function/7(medicion)  "valor real proporcionado por el modelo matematico"
  MATLAB Function/1(Wk) -> Unit Delay/1
  MATLAB Function/2(Pk) -> Unit Delay1/1
  [P2] -> MATLAB Function/3(P)
  Constant/1 -> MATLAB Function/4(R)
  Constant1/1 -> MATLAB Function/5(Q)
  H/1 -> MATLAB Function/2(H)  "Matriz H"
  Unit Delay1/1 -> [P2]  "Valor de P actualizado"
  Unit Delay/1 -> Grafica en el tiempo de w21 y w22/1, [W2], W/1  "Enviar los pesos actualizados a la red neuronal"
  Constant2/1 -> MATLAB Function/6(lambda)
  [W2] -> MATLAB Function/1(W)  "Vector de pesos"
  MATLAB Function/3(error) -> error x12/1  "error x12"

== system RHONN_EKF_FEEDBACK_FINAL_28_JULIO_2021/Subsistema de la red neuornal recurrente de alto orden (RHONN)/X3_RHONN/Sigmoidal suave1 ==
  note: Funcion sigmoidal suave S(*)
  note: Dada la ecuacion (5) del paper:
      | B > 0
      |
      | Y observado en la tesis de la Dra Alma
      | B = 2e^-3
  c : Inport
  Constante de sigmoidal suave : Constant  Value=B
  Sigmoidal suave : MATLAB Function  TreatAsAtomicUnit=on
  salida : Outport
  wires:
  Sigmoidal suave/1(sig) -> salida/1  "Señal transformada S(*)"
  c/1 -> Sigmoidal suave/2(c)  "Señal a transformar"
  Constante de sigmoidal suave/1 -> Sigmoidal suave/1(B)

== system RHONN_EKF_FEEDBACK_FINAL_28_JULIO_2021/Subsistema de la red neuornal recurrente de alto orden (RHONN)/X3_RHONN/Sigmoidal suave3 ==
  note: Funcion sigmoidal suave S(*)
  note: Dada la ecuacion (5) del paper:
      | B > 0
      |
      | Y observado en la tesis de la Dra Alma
      | B = 2e^-3
  c : Inport
  Constante de sigmoidal suave : Constant  Value=B
  Sigmoidal suave : MATLAB Function  TreatAsAtomicUnit=on
  salida : Outport
  wires:
  Sigmoidal suave/1(sig) -> salida/1  "Señal transformada S(*)"
  c/1 -> Sigmoidal suave/2(c)  "Señal a transformar"
  Constante de sigmoidal suave/1 -> Sigmoidal suave/1(B)

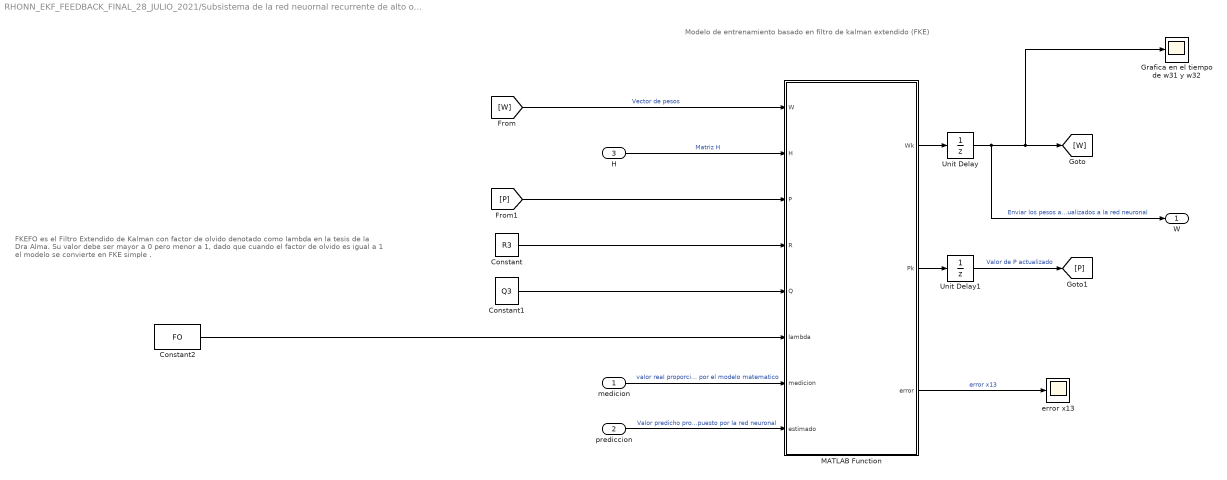
== system RHONN_EKF_FEEDBACK_FINAL_28_JULIO_2021/Subsistema de la red neuornal recurrente de alto orden (RHONN)/X3_RHONN/X3_EKF ==
  note: FKEFO es el Filtro Extendido de Kalman con factor de olvido
      |
      | denotado como lambda en la tesis de la Dra Alma.
      | Su valor debe ser mayor a 0 pero menor a 1, dado que cuando
      | el factor de olvido es igual a 1 el modelo se convierte en FKE simple .
  note: Modelo de entrenamiento basado en filtro de kalman extendido (FKE)
  medicion : Inport
  prediccion : Inport  Port=2
  H : Inport  Port=3
  Constant : Constant  Value=R3
  Constant1 : Constant  Value=Q3
  Constant2 : Constant  Value=FO
  Grafica en el tiempo de w31 y w32 : Scope
  MATLAB Function : MATLAB Function  TreatAsAtomicUnit=on
  Unit Delay : UnitDelay  InitialCondition=W3  SampleTime=-1
  Unit Delay1 : UnitDelay  InitialCondition=P3  SampleTime=-1
  error x13 : Scope
  W : Outport
  wires:
  prediccion/1 -> MATLAB Function/8(estimado)  "Valor predicho propuesto por la red neuronal"
  medicion/1 -> MATLAB Function/7(medicion)  "valor real proporcionado por el modelo matematico"
  MATLAB Function/1(Wk) -> Unit Delay/1
  [W] -> MATLAB Function/1(W)  "Vector de pesos"
  MATLAB Function/2(Pk) -> Unit Delay1/1
  [P] -> MATLAB Function/3(P)
  Constant/1 -> MATLAB Function/4(R)
  Constant1/1 -> MATLAB Function/5(Q)
  H/1 -> MATLAB Function/2(H)  "Matriz H"
  Unit Delay1/1 -> [P]  "Valor de P actualizado"
  Unit Delay/1 -> Grafica en el tiempo de w31 y w32/1, [W], W/1  "Enviar los pesos actualizados a la red neuronal"
  Constant2/1 -> MATLAB Function/6(lambda)
  MATLAB Function/3(error) -> error x13/1  "error x13"

== system RHONN_EKF_FEEDBACK_FINAL_28_JULIO_2021/Subsistema de la red neuornal recurrente de alto orden (RHONN)/X4_RHONN/Sigmoidal suave1 ==
  note: Funcion sigmoidal suave S(*)
  note: Dada la ecuacion (5) del paper:
      | B > 0
      |
      | Y observado en la tesis de la Dra Alma
      | B = 2e^-3
  c : Inport
  Constante de sigmoidal suave : Constant  Value=B
  Sigmoidal suave : MATLAB Function  TreatAsAtomicUnit=on
  salida : Outport
  wires:
  Sigmoidal suave/1(sig) -> salida/1  "Señal transformada S(*)"
  c/1 -> Sigmoidal suave/2(c)  "Señal a transformar"
  Constante de sigmoidal suave/1 -> Sigmoidal suave/1(B)

== system RHONN_EKF_FEEDBACK_FINAL_28_JULIO_2021/Subsistema de la red neuornal recurrente de alto orden (RHONN)/X4_RHONN/Sigmoidal suave2 ==
  note: Funcion sigmoidal suave S(*)
  note: Dada la ecuacion (5) del paper:
      | B > 0
      |
      | Y observado en la tesis de la Dra Alma
      | B = 2e^-3
  c : Inport
  Constante de sigmoidal suave : Constant  Value=B
  Sigmoidal suave : MATLAB Function  TreatAsAtomicUnit=on
  salida : Outport
  wires:
  Sigmoidal suave/1(sig) -> salida/1  "Señal transformada S(*)"
  c/1 -> Sigmoidal suave/2(c)  "Señal a transformar"
  Constante de sigmoidal suave/1 -> Sigmoidal suave/1(B)

== system RHONN_EKF_FEEDBACK_FINAL_28_JULIO_2021/Subsistema de la red neuornal recurrente de alto orden (RHONN)/X4_RHONN/Sigmoidal suave3 ==
  note: Funcion sigmoidal suave S(*)
  note: Dada la ecuacion (5) del paper:
      | B > 0
      |
      | Y observado en la tesis de la Dra Alma
      | B = 2e^-3
  c : Inport
  Constante de sigmoidal suave : Constant  Value=B
  Sigmoidal suave : MATLAB Function  TreatAsAtomicUnit=on
  salida : Outport
  wires:
  Sigmoidal suave/1(sig) -> salida/1  "Señal transformada S(*)"
  c/1 -> Sigmoidal suave/2(c)  "Señal a transformar"
  Constante de sigmoidal suave/1 -> Sigmoidal suave/1(B)

== system RHONN_EKF_FEEDBACK_FINAL_28_JULIO_2021/Subsistema de la red neuornal recurrente de alto orden (RHONN)/X4_RHONN/Sigmoidal suave4 ==
  note: Funcion sigmoidal suave S(*)
  note: Dada la ecuacion (5) del paper:
      | B > 0
      |
      | Y observado en la tesis de la Dra Alma
      | B = 2e^-3
  c : Inport
  Constante de sigmoidal suave : Constant  Value=B
  Sigmoidal suave : MATLAB Function  TreatAsAtomicUnit=on
  salida : Outport
  wires:
  Sigmoidal suave/1(sig) -> salida/1  "Señal transformada S(*)"
  c/1 -> Sigmoidal suave/2(c)  "Señal a transformar"
  Constante de sigmoidal suave/1 -> Sigmoidal suave/1(B)

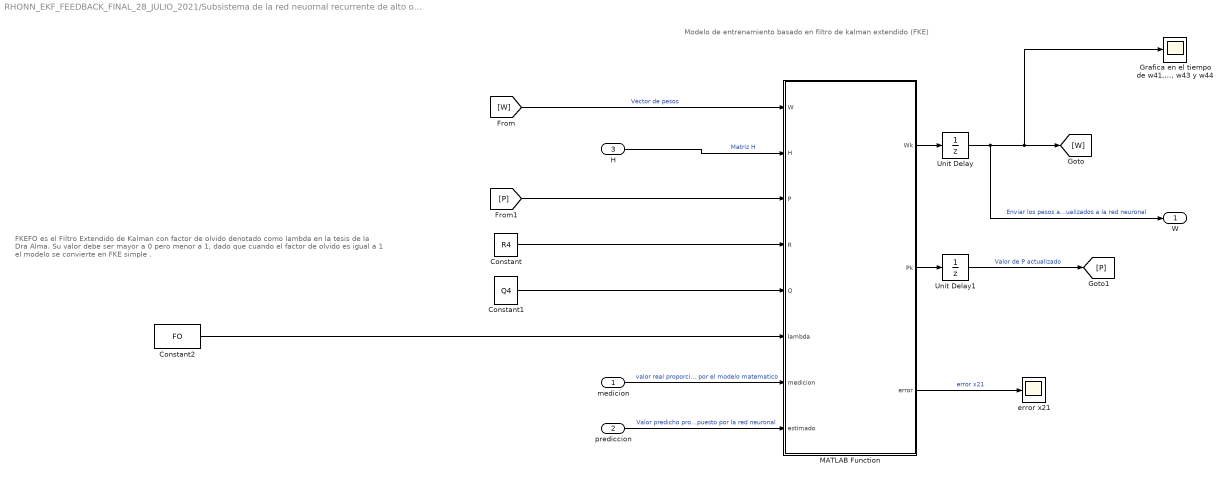
== system RHONN_EKF_FEEDBACK_FINAL_28_JULIO_2021/Subsistema de la red neuornal recurrente de alto orden (RHONN)/X4_RHONN/X4_EKF ==
  note: FKEFO es el Filtro Extendido de Kalman con factor de olvido
      |
      | denotado como lambda en la tesis de la Dra Alma.
      | Su valor debe ser mayor a 0 pero menor a 1, dado que cuando
      | el factor de olvido es igual a 1 el modelo se convierte en FKE simple .
  note: Modelo de entrenamiento basado en filtro de kalman extendido (FKE)
  medicion : Inport
  prediccion : Inport  Port=2
  H : Inport  Port=3
  Constant : Constant  Value=R4
  Constant1 : Constant  Value=Q4
  Constant2 : Constant  Value=FO
  "Grafica en el tiempo de w41, w42, w43 y w44" : Scope
  MATLAB Function : MATLAB Function  TreatAsAtomicUnit=on
  Unit Delay : UnitDelay  InitialCondition=W4  SampleTime=-1
  Unit Delay1 : UnitDelay  InitialCondition=P4  SampleTime=-1
  error x21 : Scope
  W : Outport
  wires:
  prediccion/1 -> MATLAB Function/8(estimado)  "Valor predicho propuesto por la red neuronal"
  medicion/1 -> MATLAB Function/7(medicion)  "valor real proporcionado por el modelo matematico"
  MATLAB Function/1(Wk) -> Unit Delay/1
  [W] -> MATLAB Function/1(W)  "Vector de pesos"
  MATLAB Function/2(Pk) -> Unit Delay1/1
  [P] -> MATLAB Function/3(P)
  Constant/1 -> MATLAB Function/4(R)
  Constant1/1 -> MATLAB Function/5(Q)
  H/1 -> MATLAB Function/2(H)  "Matriz H"
  Unit Delay1/1 -> [P]  "Valor de P actualizado"
  Unit Delay/1 -> "Grafica en el tiempo de w41, w42, w43 y w44"/1, [W], W/1  "Enviar los pesos actualizados a la red neuronal"
  Constant2/1 -> MATLAB Function/6(lambda)
  MATLAB Function/3(error) -> error x21/1  "error x21"

== system RHONN_EKF_FEEDBACK_FINAL_28_JULIO_2021/Subsistema de la red neuornal recurrente de alto orden (RHONN)/X5_RHONN/Sigmoidal suave1 ==
  note: Funcion sigmoidal suave S(*)
  note: Dada la ecuacion (5) del paper:
      | B > 0
      |
      | Y observado en la tesis de la Dra Alma
      | B = 2e^-3
  c : Inport
  Constante de sigmoidal suave : Constant  Value=B
  Sigmoidal suave : MATLAB Function  TreatAsAtomicUnit=on
  salida : Outport
  wires:
  Sigmoidal suave/1(sig) -> salida/1  "Señal transformada S(*)"
  c/1 -> Sigmoidal suave/2(c)  "Señal a transformar"
  Constante de sigmoidal suave/1 -> Sigmoidal suave/1(B)

== system RHONN_EKF_FEEDBACK_FINAL_28_JULIO_2021/Subsistema de la red neuornal recurrente de alto orden (RHONN)/X5_RHONN/Sigmoidal suave2 ==
  note: Funcion sigmoidal suave S(*)
  note: Dada la ecuacion (5) del paper:
      | B > 0
      |
      | Y observado en la tesis de la Dra Alma
      | B = 2e^-3
  c : Inport
  Constante de sigmoidal suave : Constant  Value=B
  Sigmoidal suave : MATLAB Function  TreatAsAtomicUnit=on
  salida : Outport
  wires:
  Sigmoidal suave/1(sig) -> salida/1  "Señal transformada S(*)"
  c/1 -> Sigmoidal suave/2(c)  "Señal a transformar"
  Constante de sigmoidal suave/1 -> Sigmoidal suave/1(B)

== system RHONN_EKF_FEEDBACK_FINAL_28_JULIO_2021/Subsistema de la red neuornal recurrente de alto orden (RHONN)/X5_RHONN/Sigmoidal suave3 ==
  note: Funcion sigmoidal suave S(*)
  note: Dada la ecuacion (5) del paper:
      | B > 0
      |
      | Y observado en la tesis de la Dra Alma
      | B = 2e^-3
  c : Inport
  Constante de sigmoidal suave : Constant  Value=B
  Sigmoidal suave : MATLAB Function  TreatAsAtomicUnit=on
  salida : Outport
  wires:
  Sigmoidal suave/1(sig) -> salida/1  "Señal transformada S(*)"
  c/1 -> Sigmoidal suave/2(c)  "Señal a transformar"
  Constante de sigmoidal suave/1 -> Sigmoidal suave/1(B)

== system RHONN_EKF_FEEDBACK_FINAL_28_JULIO_2021/Subsistema de la red neuornal recurrente de alto orden (RHONN)/X5_RHONN/Sigmoidal suave4 ==
  note: Funcion sigmoidal suave S(*)
  note: Dada la ecuacion (5) del paper:
      | B > 0
      |
      | Y observado en la tesis de la Dra Alma
      | B = 2e^-3
  c : Inport
  Constante de sigmoidal suave : Constant  Value=B
  Sigmoidal suave : MATLAB Function  TreatAsAtomicUnit=on
  salida : Outport
  wires:
  Sigmoidal suave/1(sig) -> salida/1  "Señal transformada S(*)"
  c/1 -> Sigmoidal suave/2(c)  "Señal a transformar"
  Constante de sigmoidal suave/1 -> Sigmoidal suave/1(B)

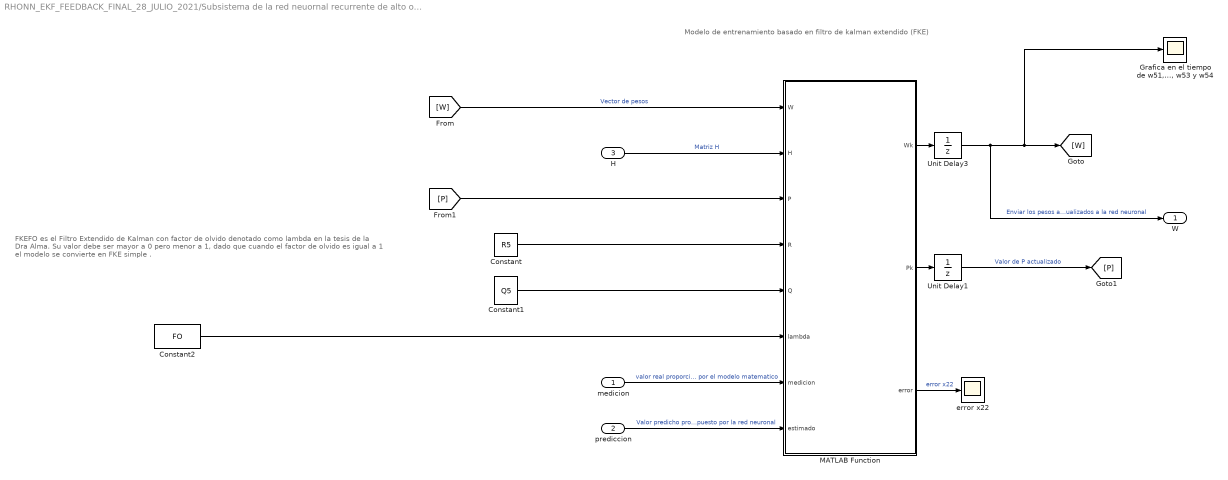
== system RHONN_EKF_FEEDBACK_FINAL_28_JULIO_2021/Subsistema de la red neuornal recurrente de alto orden (RHONN)/X5_RHONN/X5_EKF ==
  note: FKEFO es el Filtro Extendido de Kalman con factor de olvido
      |
      | denotado como lambda en la tesis de la Dra Alma.
      | Su valor debe ser mayor a 0 pero menor a 1, dado que cuando
      | el factor de olvido es igual a 1 el modelo se convierte en FKE simple .
  note: Modelo de entrenamiento basado en filtro de kalman extendido (FKE)
  medicion : Inport
  prediccion : Inport  Port=2
  H : Inport  Port=3
  Constant : Constant  Value=R5
  Constant1 : Constant  Value=Q5
  Constant2 : Constant  Value=FO
  "Grafica en el tiempo de w51, w52, w53 y w54" : Scope
  MATLAB Function : MATLAB Function  TreatAsAtomicUnit=on
  Unit Delay1 : UnitDelay  InitialCondition=P5  SampleTime=-1
  Unit Delay3 : UnitDelay  InitialCondition=W5  SampleTime=-1
  error x22 : Scope
  W : Outport
  wires:
  prediccion/1 -> MATLAB Function/8(estimado)  "Valor predicho propuesto por la red neuronal"
  medicion/1 -> MATLAB Function/7(medicion)  "valor real proporcionado por el modelo matematico"
  MATLAB Function/1(Wk) -> Unit Delay3/1
  [W] -> MATLAB Function/1(W)  "Vector de pesos"
  MATLAB Function/2(Pk) -> Unit Delay1/1
  [P] -> MATLAB Function/3(P)
  Constant/1 -> MATLAB Function/4(R)
  Constant1/1 -> MATLAB Function/5(Q)
  H/1 -> MATLAB Function/2(H)  "Matriz H"
  Unit Delay1/1 -> [P]  "Valor de P actualizado"
  Unit Delay3/1 -> "Grafica en el tiempo de w51, w52, w53 y w54"/1, [W], W/1  "Enviar los pesos actualizados a la red neuronal"
  Constant2/1 -> MATLAB Function/6(lambda)
  MATLAB Function/3(error) -> error x22/1  "error x22"

== system RHONN_EKF_FEEDBACK_FINAL_28_JULIO_2021/Subsistema de la red neuornal recurrente de alto orden (RHONN)/X6_RHONN/Sigmoidal suave1 ==
  note: Funcion sigmoidal suave S(*)
  note: Dada la ecuacion (5) del paper:
      | B > 0
      |
      | Y observado en la tesis de la Dra Alma
      | B = 2e^-3
  c : Inport
  Constante de sigmoidal suave : Constant  Value=B
  Sigmoidal suave : MATLAB Function  TreatAsAtomicUnit=on
  salida : Outport
  wires:
  Sigmoidal suave/1(sig) -> salida/1  "Señal transformada S(*)"
  c/1 -> Sigmoidal suave/2(c)  "Señal a transformar"
  Constante de sigmoidal suave/1 -> Sigmoidal suave/1(B)

== system RHONN_EKF_FEEDBACK_FINAL_28_JULIO_2021/Subsistema de la red neuornal recurrente de alto orden (RHONN)/X6_RHONN/Sigmoidal suave2 ==
  note: Funcion sigmoidal suave S(*)
  note: Dada la ecuacion (5) del paper:
      | B > 0
      |
      | Y observado en la tesis de la Dra Alma
      | B = 2e^-3
  c : Inport
  Constante de sigmoidal suave : Constant  Value=B
  Sigmoidal suave : MATLAB Function  TreatAsAtomicUnit=on
  salida : Outport
  wires:
  Sigmoidal suave/1(sig) -> salida/1  "Señal transformada S(*)"
  c/1 -> Sigmoidal suave/2(c)  "Señal a transformar"
  Constante de sigmoidal suave/1 -> Sigmoidal suave/1(B)

== system RHONN_EKF_FEEDBACK_FINAL_28_JULIO_2021/Subsistema de la red neuornal recurrente de alto orden (RHONN)/X6_RHONN/Sigmoidal suave3 ==
  note: Funcion sigmoidal suave S(*)
  note: Dada la ecuacion (5) del paper:
      | B > 0
      |
      | Y observado en la tesis de la Dra Alma
      | B = 2e^-3
  c : Inport
  Constante de sigmoidal suave : Constant  Value=B
  Sigmoidal suave : MATLAB Function  TreatAsAtomicUnit=on
  salida : Outport
  wires:
  Sigmoidal suave/1(sig) -> salida/1  "Señal transformada S(*)"
  c/1 -> Sigmoidal suave/2(c)  "Señal a transformar"
  Constante de sigmoidal suave/1 -> Sigmoidal suave/1(B)

== system RHONN_EKF_FEEDBACK_FINAL_28_JULIO_2021/Subsistema de la red neuornal recurrente de alto orden (RHONN)/X6_RHONN/Sigmoidal suave4 ==
  note: Funcion sigmoidal suave S(*)
  note: Dada la ecuacion (5) del paper:
      | B > 0
      |
      | Y observado en la tesis de la Dra Alma
      | B = 2e^-3
  c : Inport
  Constante de sigmoidal suave : Constant  Value=B
  Sigmoidal suave : MATLAB Function  TreatAsAtomicUnit=on
  salida : Outport
  wires:
  Sigmoidal suave/1(sig) -> salida/1  "Señal transformada S(*)"
  c/1 -> Sigmoidal suave/2(c)  "Señal a transformar"
  Constante de sigmoidal suave/1 -> Sigmoidal suave/1(B)

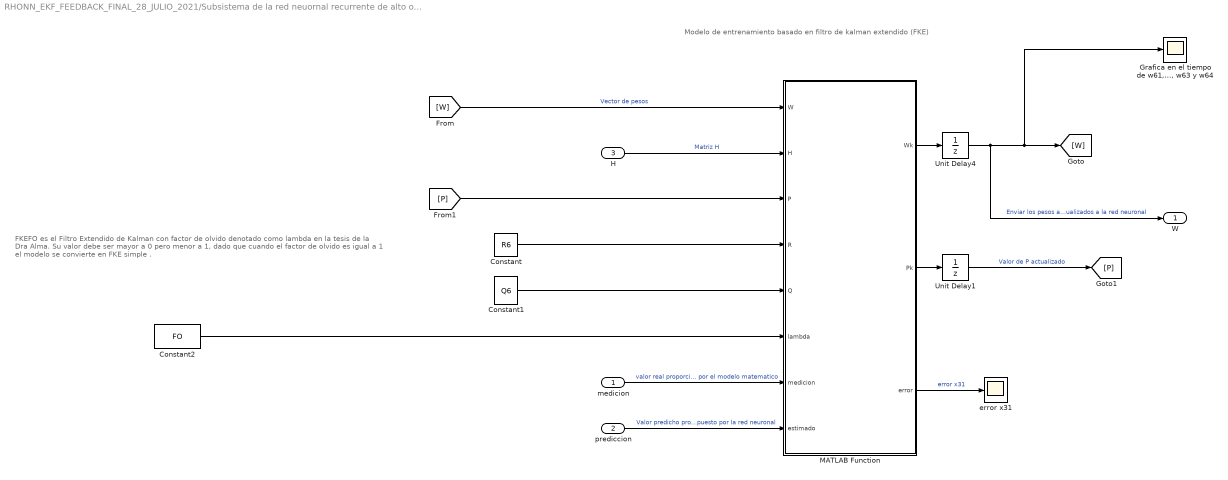
== system RHONN_EKF_FEEDBACK_FINAL_28_JULIO_2021/Subsistema de la red neuornal recurrente de alto orden (RHONN)/X6_RHONN/X6_EKF ==
  note: FKEFO es el Filtro Extendido de Kalman con factor de olvido
      |
      | denotado como lambda en la tesis de la Dra Alma.
      | Su valor debe ser mayor a 0 pero menor a 1, dado que cuando
      | el factor de olvido es igual a 1 el modelo se convierte en FKE simple .
  note: Modelo de entrenamiento basado en filtro de kalman extendido (FKE)
  medicion : Inport
  prediccion : Inport  Port=2
  H : Inport  Port=3
  Constant : Constant  Value=R6
  Constant1 : Constant  Value=Q6
  Constant2 : Constant  Value=FO
  "Grafica en el tiempo de w61, w62, w63 y w64" : Scope
  MATLAB Function : MATLAB Function  TreatAsAtomicUnit=on
  Unit Delay1 : UnitDelay  InitialCondition=P6  SampleTime=-1
  Unit Delay4 : UnitDelay  InitialCondition=W6  SampleTime=-1
  error x31 : Scope
  W : Outport
  wires:
  prediccion/1 -> MATLAB Function/8(estimado)  "Valor predicho propuesto por la red neuronal"
  medicion/1 -> MATLAB Function/7(medicion)  "valor real proporcionado por el modelo matematico"
  MATLAB Function/1(Wk) -> Unit Delay4/1
  [W] -> MATLAB Function/1(W)  "Vector de pesos"
  MATLAB Function/2(Pk) -> Unit Delay1/1
  [P] -> MATLAB Function/3(P)
  Constant/1 -> MATLAB Function/4(R)
  Constant1/1 -> MATLAB Function/5(Q)
  H/1 -> MATLAB Function/2(H)  "Matriz H"
  Unit Delay1/1 -> [P]  "Valor de P actualizado"
  Unit Delay4/1 -> "Grafica en el tiempo de w61, w62, w63 y w64"/1, [W], W/1  "Enviar los pesos actualizados a la red neuronal"
  Constant2/1 -> MATLAB Function/6(lambda)
  MATLAB Function/3(error) -> error x31/1  "error x31"

== system RHONN_EKF_FEEDBACK_FINAL_28_JULIO_2021/Subsistema de la red neuornal recurrente de alto orden (RHONN)/X7_RHONN/Sigmoidal suave1 ==
  note: Funcion sigmoidal suave S(*)
  note: Dada la ecuacion (5) del paper:
      | B > 0
      |
      | Y observado en la tesis de la Dra Alma
      | B = 2e^-3
  c : Inport
  Constante de sigmoidal suave : Constant  Value=B
  Sigmoidal suave : MATLAB Function  TreatAsAtomicUnit=on
  salida : Outport
  wires:
  Sigmoidal suave/1(sig) -> salida/1  "Señal transformada S(*)"
  c/1 -> Sigmoidal suave/2(c)  "Señal a transformar"
  Constante de sigmoidal suave/1 -> Sigmoidal suave/1(B)

== system RHONN_EKF_FEEDBACK_FINAL_28_JULIO_2021/Subsistema de la red neuornal recurrente de alto orden (RHONN)/X7_RHONN/Sigmoidal suave2 ==
  note: Funcion sigmoidal suave S(*)
  note: Dada la ecuacion (5) del paper:
      | B > 0
      |
      | Y observado en la tesis de la Dra Alma
      | B = 2e^-3
  c : Inport
  Constante de sigmoidal suave : Constant  Value=B
  Sigmoidal suave : MATLAB Function  TreatAsAtomicUnit=on
  salida : Outport
  wires:
  Sigmoidal suave/1(sig) -> salida/1  "Señal transformada S(*)"
  c/1 -> Sigmoidal suave/2(c)  "Señal a transformar"
  Constante de sigmoidal suave/1 -> Sigmoidal suave/1(B)

== system RHONN_EKF_FEEDBACK_FINAL_28_JULIO_2021/Subsistema de la red neuornal recurrente de alto orden (RHONN)/X7_RHONN/Sigmoidal suave3 ==
  note: Funcion sigmoidal suave S(*)
  note: Dada la ecuacion (5) del paper:
      | B > 0
      |
      | Y observado en la tesis de la Dra Alma
      | B = 2e^-3
  c : Inport
  Constante de sigmoidal suave : Constant  Value=B
  Sigmoidal suave : MATLAB Function  TreatAsAtomicUnit=on
  salida : Outport
  wires:
  Sigmoidal suave/1(sig) -> salida/1  "Señal transformada S(*)"
  c/1 -> Sigmoidal suave/2(c)  "Señal a transformar"
  Constante de sigmoidal suave/1 -> Sigmoidal suave/1(B)

== system RHONN_EKF_FEEDBACK_FINAL_28_JULIO_2021/Subsistema de la red neuornal recurrente de alto orden (RHONN)/X7_RHONN/Sigmoidal suave4 ==
  note: Funcion sigmoidal suave S(*)
  note: Dada la ecuacion (5) del paper:
      | B > 0
      |
      | Y observado en la tesis de la Dra Alma
      | B = 2e^-3
  c : Inport
  Constante de sigmoidal suave : Constant  Value=B
  Sigmoidal suave : MATLAB Function  TreatAsAtomicUnit=on
  salida : Outport
  wires:
  Sigmoidal suave/1(sig) -> salida/1  "Señal transformada S(*)"
  c/1 -> Sigmoidal suave/2(c)  "Señal a transformar"
  Constante de sigmoidal suave/1 -> Sigmoidal suave/1(B)
